simulink model "Ex_2_Bidirectional_drive_with_H_bridge"  (R2020a)
settings: Solver=FixedStepAuto  StartTime=0.0  StopTime=8  FixedStep=0.001  RelTol=1e-3
values from neighbouring files (symbols this model uses):
  J = 0.005    [motor_parameters.mat]
  Ke = 2.3    [motor_parameters.mat]
  Kf = 0.3    [motor_parameters.mat]
  Kt = 2.19    [motor_parameters.mat]
  L = 1    [motor_parameters.mat]
  R = 1.1    [motor_parameters.mat]
libraries: fl_lib x7, ee_lib x6, nesl_utility x5
settings Model: Creator=alexr  LastModifiedBy=alexr

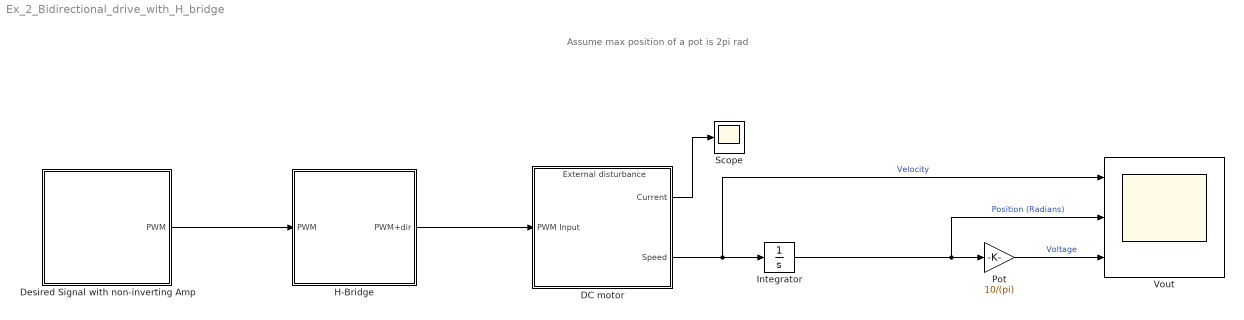
== system Ex_2_Bidirectional_drive_with_H_bridge ==
  note: Assume max position of a pot is 2pi rad
  DC motor : Subsystem
      settings: PortSchema="{\"entries\":[{\"content\":{\"sides\":[{\"content\":{\"connectorIds\":[\"In1\"]},\"type\":\"ConnectorPlacement.EquallySpacedRectSide\",\"uuid\":\"b8964f03-f732-4eca-8bb3-271c6a142913\"},{\"content\":{\"connectorIds\":[\"Out1\",\"Out2\"],\"side\":\"RIGHT\"},\"type\":\"ConnectorPlacement.EquallySpacedRectSide\",\"uuid\":\"d9454742-672e-4fe5-95f0-bbd13d54c419\"},{\"content\":{\"connectorIds\":[\"In2\"],\"side\":\"TOP\"},\"type\":\"ConnectorPlacement.EquallySpacedRectSide\",\"uuid\":\"e6caae02-41c3-4a6e-bc88-5a1dbae17927\"}]},\"type\":\"ConnectorPlacement.EquallySpacedConnector\",\"uuid\":\"63b5fd96-b4f9-40de-b12b-448e4637e2c5\"}],\"packageUris\":[\"http://schema.mathworks.com/mf0/Connector/19700101\"],\"version\":\"1.0\"}"
  Desired Signal with non-inverting Amp : Subsystem
  H-Bridge : Subsystem
  Integrator : Integrator
  Pot : Gain  Gain=10/(pi)
  Scope : Scope
  Vout : Scope  NumInputPorts=3
  wires:
  Integrator/1 -> Vout/2, Pot/1  "Position (Radians)"
  Pot/1 -> Vout/3  "Voltage"
  DC motor/1(Current) -> Scope/1
  DC motor/2(Speed) -> Vout/1, Integrator/1  "Velocity"
  Desired Signal with non-inverting Amp/1(PWM) -> H-Bridge/1(PWM)
  H-Bridge/1(PWM+dir) -> DC motor/1(PWM Input)

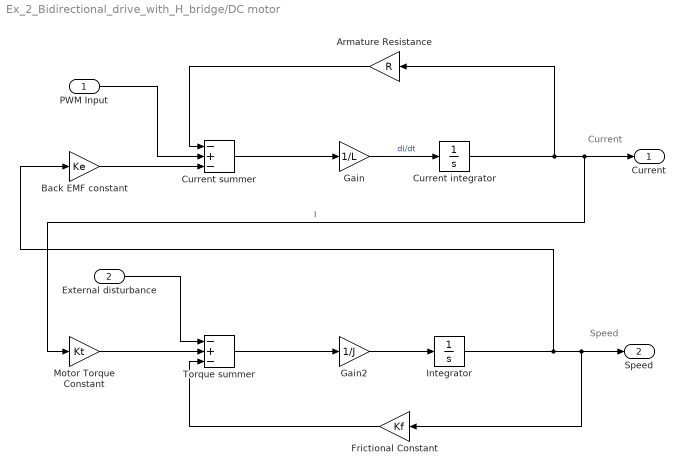
== system Ex_2_Bidirectional_drive_with_H_bridge/DC motor ==
  note: Speed
  note: Current
  PWM Input : Inport
  External disturbance : Inport  Port=2
  Armature Resistance : Gain  Gain=R
  Back EMF constant : Gain  Gain=Ke
  Current integrator : Integrator
  Current summer : Sum  Inputs=-+-
  Frictional Constant : Gain  Gain=Kf
  Gain : Gain  Gain=1/L
  Gain2 : Gain  Gain=1/J
  Integrator : Integrator
  Motor Torque Constant : Gain  Gain=Kt
  Torque summer : Sum  Inputs=-+-
  Current : Outport
  Speed : Outport  Port=2
  wires:
  Current summer/1 -> Gain/1
  Gain2/1 -> Integrator/1
  Integrator/1 -> Back EMF constant/1, Speed/1, Frictional Constant/1
  Torque summer/1 -> Gain2/1
  Armature Resistance/1 -> Current summer/1
  PWM Input/1 -> Current summer/2
  Gain/1 -> Current integrator/1  "di/dt"
  Motor Torque Constant/1 -> Torque summer/2
  External disturbance/1 -> Torque summer/1
  Frictional Constant/1 -> Torque summer/3
  Current integrator/1 -> Armature Resistance/1, Current/1, Motor Torque Constant/1  "I"
  Back EMF constant/1 -> Current summer/3

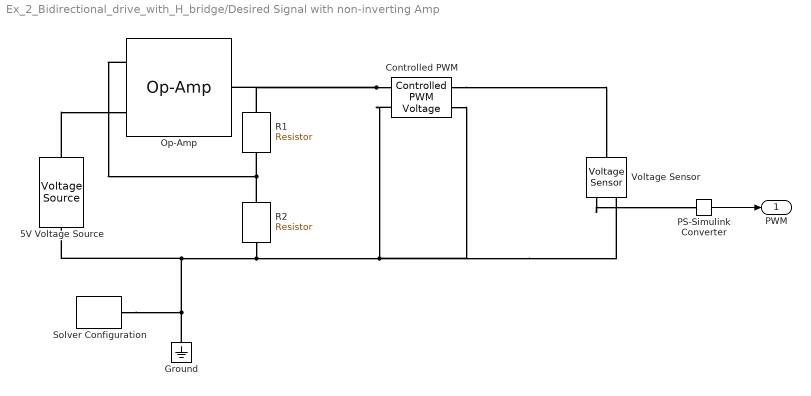
== system Ex_2_Bidirectional_drive_with_H_bridge/Desired Signal with non-inverting Amp ==
  "5V Voltage Source " : ee_lib/Sources/Voltage Source  dc_voltage=5 V  ac_voltage=0 V  ac_shift=0 rad  ac_frequency=60 Hz  noise_mode=0  PSD=0 V^2/Hz  repeatability=1  auto_seed=983448592  user_seed=0  sample_time=1e-3 s  i_specify=off  i_priority=None  i=0 A  i_nominal_specify=off  i_nominal_unit=A  i_nominal_value=1  v_specify=off  v_priority=None  v=0 V  v_nominal_specify=off  v_nominal_unit=V  v_nominal_value=1
  "Controlled PWM " : ee_lib/Integrated Circuits/Controlled PWM Voltage  F=4000 Hz  TD=0 s  pulse_width_offset=0 s  pulse_min=0 s  Vmin=0 V  Vmax=10 V  Vm=10 V  pwm_or_av=2  event_type=1  sample_time=1e-6 s  u_min=0  u_max=5
  "Ground " : fl_lib/Electrical/Electrical Elements/Electrical Reference
      settings: SourceProductBaseCode=MT,SS
  "Op-Amp " : fl_lib/Electrical/Electrical Elements/Op-Amp  outI_specify=off  outI_priority=None  outI=0 A  outI_nominal_specify=off  outI_nominal_unit=A  outI_nominal_value=1
  PS-Simulink Converter : nesl_utility/PS-Simulink Converter  PhysicalDomain=network_engine_domain  SubClassName=ps_output  LeftPortType=input  RightPortType=output  PseudoPeriodic=off  Frequencies=[]  Unit=inherit  AffineConversion=off
  R1 : ee_lib/Passive/Resistor  R=1000 Ohm  R_tol=5  enable_R_tol=0  tol_distribution=1  nSigma=4  enable_operating_limits=0  operating_limit_action=2  max_working_voltage=100 V  power_rating=1 W  enable_faults=0  fault_action=1  R_faulted=inf Ohm  enable_temporal_fault=0  t_fault=1 s  enable_behavioral_fault=0  max_permissible_current=1 A  t_fail_on_current=1 s  noise_mode=0  sample_time=1e-3 s  repeatability=1  auto_seed=3922754097  user_seed=0  Tdevice=25 degC  alpha=3.93e-3 1/K  Tmeas=25 degC  thermal_mass=100 J/K  power_derating_T1=70 degC  power_derating_T2=155 degC  operating_temperature_range_vec=[-50, 150] degC  temperature_specify=off  temperature_priority=High  temperature=298.15 K  temperature_nominal_specify=off  temperature_nominal_unit=K  temperature_nominal_value=1
  R2 : ee_lib/Passive/Resistor  R=1000 Ohm  R_tol=5  enable_R_tol=0  tol_distribution=1  nSigma=4  enable_operating_limits=0  operating_limit_action=2  max_working_voltage=100 V  power_rating=1 W  enable_faults=0  fault_action=1  R_faulted=inf Ohm  enable_temporal_fault=0  t_fault=1 s  enable_behavioral_fault=0  max_permissible_current=1 A  t_fail_on_current=1 s  noise_mode=0  sample_time=1e-3 s  repeatability=1  auto_seed=654458608  user_seed=0  Tdevice=25 degC  alpha=3.93e-3 1/K  Tmeas=25 degC  thermal_mass=100 J/K  power_derating_T1=70 degC  power_derating_T2=155 degC  operating_temperature_range_vec=[-50, 150] degC  temperature_specify=off  temperature_priority=High  temperature=298.15 K  temperature_nominal_specify=off  temperature_nominal_unit=K  temperature_nominal_value=1
  "Solver Configuration " : nesl_utility/Solver Configuration  PhysicalDomain=network_engine_domain  SubClassName=solver  LeftPortType=input  RightPortType=generic  Tones=[]  Harmonics=[]  SimulateNoise=off  Profile=off  UseLocalSampling=off  EnableSwitchedLinearOptims=on  FrequencyDomain=off  UseCCode=off  RelTol=0.001  AbsTol=1e-06  MinStep=1e-09  ToWorkspace=off  RevertToSquareIcSolve=off  NumHomotopyIterations=100  PhasorMode=off  PhasorModeNumHarmonics=1  DoDC=off  ResidualTolerance=1e-09  UseLocalSolver=off  LocalSolverChoice=NE_BACKWARD_EULER_ADVANCER  LocalSolverSampleTime=0.001  DoFixedCost=off  MaxNonlinIter=3  MaxModeIter=2  LinearAlgebra=auto  EquationFormulation=NE_TIME_EF  DelaysMemoryBudget=1024  AutomaticFiltering=on  FilteringTimeConstant=0.001  PartitionStorageMethod=AS_NEEDED  PartitionMemoryBudget=1024  PartitionMethod=ROBUST
  Voltage Sensor : fl_lib/Electrical/Electrical Sensors/Voltage Sensor
  PWM : Outport
  wires:
  PS-Simulink Converter/1 -> PWM/1
  connections:
  R2/LConn1 -- "Op-Amp "/LConn2 -- R1/RConn1
  "Controlled PWM "/LConn1 -- "Op-Amp "/RConn1 -- R1/LConn1
  "Solver Configuration "/RConn1 -- "Ground "/LConn1 -- R2/RConn1 -- Voltage Sensor/RConn2 -- "Controlled PWM "/RConn2 -- "Controlled PWM "/LConn2 -- "5V Voltage Source "/RConn1
  "5V Voltage Source "/LConn1 -- "Op-Amp "/LConn1
  "Controlled PWM "/RConn1 -- Voltage Sensor/LConn1
  Voltage Sensor/RConn1 -- PS-Simulink Converter/LConn1

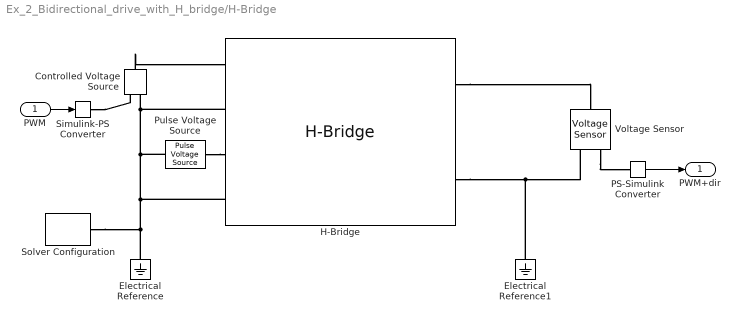
== system Ex_2_Bidirectional_drive_with_H_bridge/H-Bridge ==
  PWM : Inport
  Controlled Voltage Source : fl_lib/Electrical/Electrical Sources/Controlled Voltage Source
  Electrical Reference : fl_lib/Electrical/Electrical Elements/Electrical Reference
      settings: SourceProductBaseCode=MT,SS
  Electrical Reference1 : fl_lib/Electrical/Electrical Elements/Electrical Reference
      settings: SourceProductBaseCode=MT,SS
  H-Bridge : ee_lib/Semiconductors & Converters/Converters/H-Bridge  supply_ports=ee.enum.supply_ports.hidesupply  Venable=0.1 V  Vmax=10 V  Vreverse=2.5 V  Vbrake=10 V  Vm=10 V  pwm_or_av=ee.enum.pwm_or_av.averaged  regenerative_braking_mode=ee.enum.converters.regenerative_braking_mode.always_enabled  discontinuous=ee.enum.current_profile.continuous  freewheeling_mode=ee.enum.converters.freewheeling_mode.one_switch_one_diode  Ron=0.1 Ohm  Don=0.05 Ohm  Goff=1e-6 S  Rload=10 Ohm  Lload=1e-5 H  F=10 kHz  thermal_mass=100 J/K  initial_temperature=298.15 K  Ron2=0.1 Ohm  Don2=0.05 Ohm  Tmeas=298.15 K  Tmeas2=398.15 K
  PS-Simulink Converter : nesl_utility/PS-Simulink Converter  PhysicalDomain=network_engine_domain  SubClassName=ps_output  LeftPortType=input  RightPortType=output  PseudoPeriodic=off  Frequencies=[]  Unit=inherit  AffineConversion=off
  "Pulse Voltage Source " : ee_lib/Additional Components/SPICE Sources/Pulse Voltage Source  V1=0 V  V2=5 V  TD=1 s  TR=1e-9 s  TF=1e-9 s  PW=1 s  PER=2 s
      settings: SourceProductBaseCode=PS  InternalSimscapePortConfiguration="{\"Bottom\":[],\"Left\":[{\"id\":\"p\",\"label\":\"\",\"type\":\"foundation.electrical.electrical\"}],\"Right\":[{\"id\":\"n\",\"label\":\"\",\"type\":\"foundation.electrical.electrical\"}],\"Top\":[]}"
  Simulink-PS Converter : nesl_utility/Simulink-PS Converter  PhysicalDomain=network_engine_domain  SubClassName=ps_input  LeftPortType=input  RightPortType=output  PseudoPeriodic=off  Frequencies=[]  NoiseDistribution=none  NoiseParameters=[]  Unit=1  AffineConversion=off  FilteringAndDerivatives=provide  SimscapeFilterOrder=1  InputFilterTimeConstant=0.001  UdotUserProvided=0
  Solver Configuration : nesl_utility/Solver Configuration  PhysicalDomain=network_engine_domain  SubClassName=solver  LeftPortType=input  RightPortType=generic  Tones=[]  Harmonics=[]  SimulateNoise=off  Profile=off  UseLocalSampling=off  EnableSwitchedLinearOptims=on  FrequencyDomain=off  UseCCode=off  RelTol=0.001  AbsTol=1e-06  MinStep=1e-09  ToWorkspace=off  RevertToSquareIcSolve=off  NumHomotopyIterations=100  PhasorMode=off  PhasorModeNumHarmonics=1  DoDC=off  ResidualTolerance=1e-09  UseLocalSolver=off  LocalSolverChoice=NE_BACKWARD_EULER_ADVANCER  LocalSolverSampleTime=0.001  DoFixedCost=off  MaxNonlinIter=3  MaxModeIter=2  LinearAlgebra=auto  EquationFormulation=NE_TIME_EF  DelaysMemoryBudget=1024  AutomaticFiltering=on  FilteringTimeConstant=0.001  PartitionStorageMethod=AS_NEEDED  PartitionMemoryBudget=1024  PartitionMethod=ROBUST
  Voltage Sensor : fl_lib/Electrical/Electrical Sensors/Voltage Sensor
  PWM+dir : Outport
  wires:
  PS-Simulink Converter/1 -> PWM+dir/1
  PWM/1 -> Simulink-PS Converter/1
  connections:
  Controlled Voltage Source/LConn1 -- H-Bridge/LConn1
  Electrical Reference/LConn1 -- Solver Configuration/RConn1 -- H-Bridge/LConn4 -- "Pulse Voltage Source "/RConn1 -- H-Bridge/LConn2 -- Controlled Voltage Source/RConn2
  "Pulse Voltage Source "/LConn1 -- H-Bridge/LConn3
  H-Bridge/RConn1 -- Voltage Sensor/LConn1
  Voltage Sensor/RConn1 -- PS-Simulink Converter/LConn1
  Simulink-PS Converter/RConn1 -- Controlled Voltage Source/RConn1
  H-Bridge/RConn2 -- Electrical Reference1/LConn1 -- Voltage Sensor/RConn2
